simulink library "Pressure_Drop"  (R2018b)
settings: Solver=ode45  StartTime=0.0  StopTime=10.0  RelTol=1e-3  EnableMultiTasking=on
undefined symbols (not defined in the file): DPConstant, DPLinear, DPQuadratic, Pressure
libraries: simulink x1
settings Model: Creator=lena.frank  LastModifiedBy=drhf
settings DataIOCC: LimitDataPoints=on  SaveFormat=Array  SignalLoggingSaveFormat=ModelDataLogs
settings OptimizationCC: ExpressionDepthLimit=2147483647  LifeSpan=inf
settings DebuggingCC: UnderspecifiedInitializationDetection=Classic  MergeDetectMultiDrivingBlocksExec=none  SolverPrmCheckMsg=warning  FcnCallInpInsideContextMsg=warning  StateNameClashWarn=warning  SFUnexpectedBacktrackingDiag=warning  SFNoUnconditionalDefaultTransitionDiag=warning  SFExecutionAtInitializationDiag=none
settings HardwareCC: ProdBitPerPointer=32  ProdBitPerSizeT=32  ProdBitPerPtrDiffT=32  ProdLargestAtomicFloat=None  ProdIntDivRoundTo=Undefined  ProdEndianess=Unspecified  ProdWordSize=32  ProdHWDeviceType=32-bit Generic
settings ModelReferenceCC: PropagateSignalLabelsOutOfModel=off
settings SFSimCC: SimUseLocalCustomCode=off
settings RTWCC: RTWUseLocalCustomCode=off
settings CodeAppCC: StateflowObjectComments=on
settings GRTTargetCC: TargetLangStandard=C89/C90 (ANSI)  GeneratePreprocessorConditionals=Disable all  CombineOutputUpdateFcns=off  GRTInterface=on
settings ConfigComp: CovMetricSettings=dw  CovHtmlReporting=on  CovSaveCumulativeToWorkspaceVar=on  CovSaveSingleToWorkspaceVar=on  CovExternalEMLEnable=off

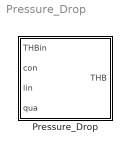
== system Pressure_Drop ==
  Pressure_Drop : Subsystem  mask(pressure drop){}
      mask help:
      | Pressure drop according to input values of con, lin and qua:
      | dp = con + lin*mdot + qua*mdot²
      | The coefficients are also added to the correponding THB elements.
      mask Help: web(fullfile(path_carnot('help'),'Pressure_Drop.html'),'-helpbrowser')

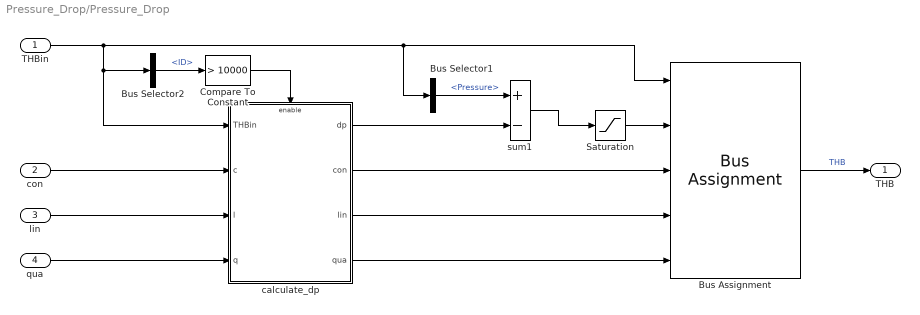
== system Pressure_Drop/Pressure_Drop ==
  THBin : Inport
  con : Inport  Port=2
  lin : Inport  Port=3
  qua : Inport  Port=4
  Bus Assignment : BusAssignment  AssignedSignals=Pressure,DPConstant,DPLinear,DPQuadratic
  Bus Selector1 : BusSelector  OutputSignals=Pressure
  Bus Selector2 : BusSelector  OutputSignals=ID
  Compare To Constant : simulink/Logic and Bit Operations/Compare To Constant  relop=>  const=10000  OutDataTypeStr=boolean
  Saturation : Saturate  UpperLimit=inf  LowerLimit=0
  calculate_dp : Subsystem
  sum1 : Sum  Inputs=+-  SaturateOnIntegerOverflow=on  InputSameDT=on  OutDataTypeStr=Inherit: Same as first input
  THB : Outport
  wires:
  THBin/1 -> Bus Selector2/1, calculate_dp/1(THBin), Bus Assignment/1, Bus Selector1/1
  sum1/1 -> Saturation/1
  Bus Assignment/1 -> THB/1  "THB"
  Bus Selector1/1 -> sum1/1  "<Pressure>"
  Saturation/1 -> Bus Assignment/2
  con/1 -> calculate_dp/2(c)
  lin/1 -> calculate_dp/3(l)
  qua/1 -> calculate_dp/4(q)
  calculate_dp/2(con) -> Bus Assignment/3
  calculate_dp/3(lin) -> Bus Assignment/4
  calculate_dp/4(qua) -> Bus Assignment/5
  calculate_dp/1(dp) -> sum1/2
  Compare To Constant/1 -> calculate_dp/Enable
  Bus Selector2/1 -> Compare To Constant/1  "<ID>"

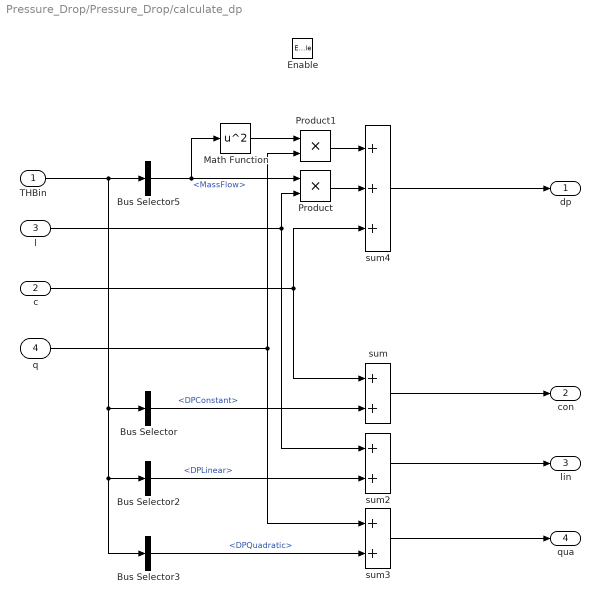
== system Pressure_Drop/Pressure_Drop/calculate_dp ==
  THBin : Inport
  c : Inport  Port=2
  l : Inport  Port=3
  q : Inport  Port=4
  Enable : EnablePort
  Bus Selector : BusSelector  OutputSignals=DPConstant
  Bus Selector2 : BusSelector  OutputSignals=DPLinear
  Bus Selector3 : BusSelector  OutputSignals=DPQuadratic
  Bus Selector5 : BusSelector  OutputSignals=MassFlow
  Math Function : Math  Operator=square  SaturateOnIntegerOverflow=on
  Product : Product
  Product1 : Product
  sum : Sum  SaturateOnIntegerOverflow=on  InputSameDT=on  OutDataTypeStr=Inherit: Same as first input
  sum2 : Sum  SaturateOnIntegerOverflow=on  InputSameDT=on  OutDataTypeStr=Inherit: Same as first input
  sum3 : Sum  SaturateOnIntegerOverflow=on  InputSameDT=on  OutDataTypeStr=Inherit: Same as first input
  sum4 : Sum  Inputs=3  SaturateOnIntegerOverflow=on  InputSameDT=on  OutDataTypeStr=Inherit: Same as first input
  dp : Outport
  con : Outport  Port=2
  lin : Outport  Port=3
  qua : Outport  Port=4
  wires:
  q/1 -> sum3/1, Product1/2
  c/1 -> sum/1, sum4/3
  l/1 -> sum2/1, Product/2
  THBin/1 -> Bus Selector5/1, Bus Selector3/1, Bus Selector2/1, Bus Selector/1
  Bus Selector5/1 -> Math Function/1, Product/1  "<MassFlow>"
  sum4/1 -> dp/1
  Math Function/1 -> Product1/1
  Bus Selector3/1 -> sum3/2  "<DPQuadratic>"
  Bus Selector/1 -> sum/2  "<DPConstant>"
  Bus Selector2/1 -> sum2/2  "<DPLinear>"
  Product1/1 -> sum4/1
  Product/1 -> sum4/2
  sum/1 -> con/1
  sum2/1 -> lin/1
  sum3/1 -> qua/1
